simulink library "csu_gyk_gyro_kinematics_lib"  (R2014b)
settings: Solver=ode45  SolverMode=SingleTasking  StartTime=0.0  StopTime=10.0  RelTol=1e-3
undefined symbols (not defined in the file or in its folder): gyk_miru_gyro_dcm
libraries: util_info_lib x1
settings Model: Creator=hcannon  LastModifiedBy=mstewart

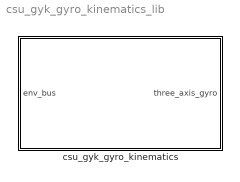
== system csu_gyk_gyro_kinematics_lib ==
  csu_gyk_gyro_kinematics : Subsystem

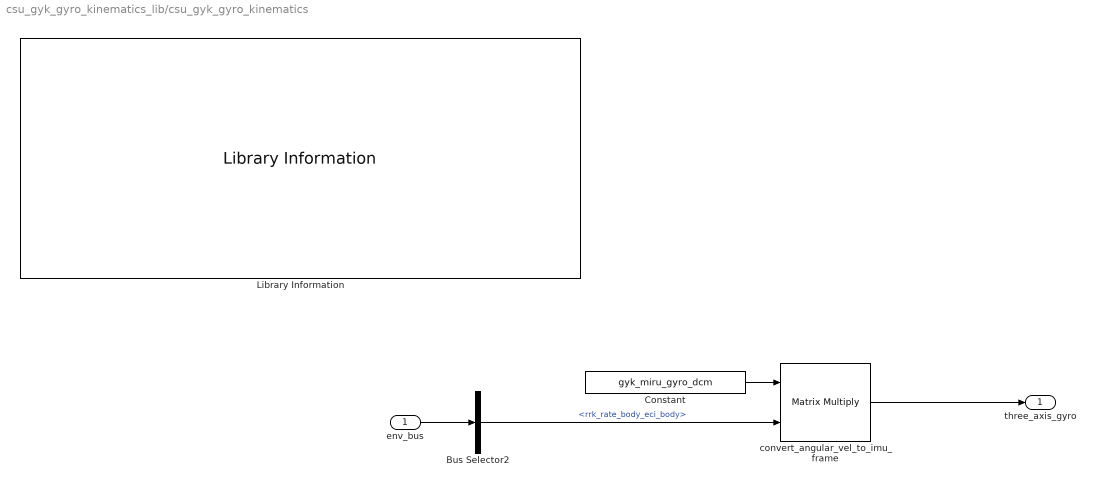
== system csu_gyk_gyro_kinematics_lib/csu_gyk_gyro_kinematics ==
  env_bus : Inport
  Bus Selector2 : BusSelector  OutputSignals=lander_state_bus.rrk_rate_body_eci_body
  Constant : Constant  Value=gyk_miru_gyro_dcm
  Library Information : util_info_lib/Library Information  owner='escrane'
  convert_angular_vel_to_imu_frame : Product  Multiplication=Matrix(*)  RndMeth=Zero
  three_axis_gyro : Outport
  wires:
  env_bus/1 -> Bus Selector2/1
  Constant/1 -> convert_angular_vel_to_imu_frame/1
  Bus Selector2/1 -> convert_angular_vel_to_imu_frame/2  "<rrk_rate_body_eci_body>"
  convert_angular_vel_to_imu_frame/1 -> three_axis_gyro/1
